simulink model "mc_sevcong4s10"  (R2025a)
settings: Solver=FixedStepAuto  StartTime=0.0  StopTime=10.0  FixedStep=0.05  RelTol=1e-3
settings Model: Creator=adam  LastModifiedBy=adam

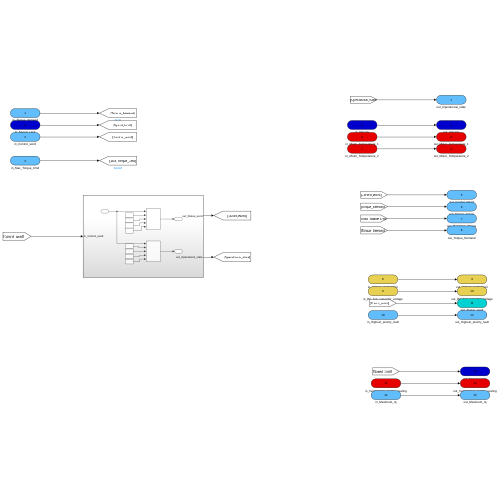
[thumbnail: Simulink's stored preview of the top-level diagram]
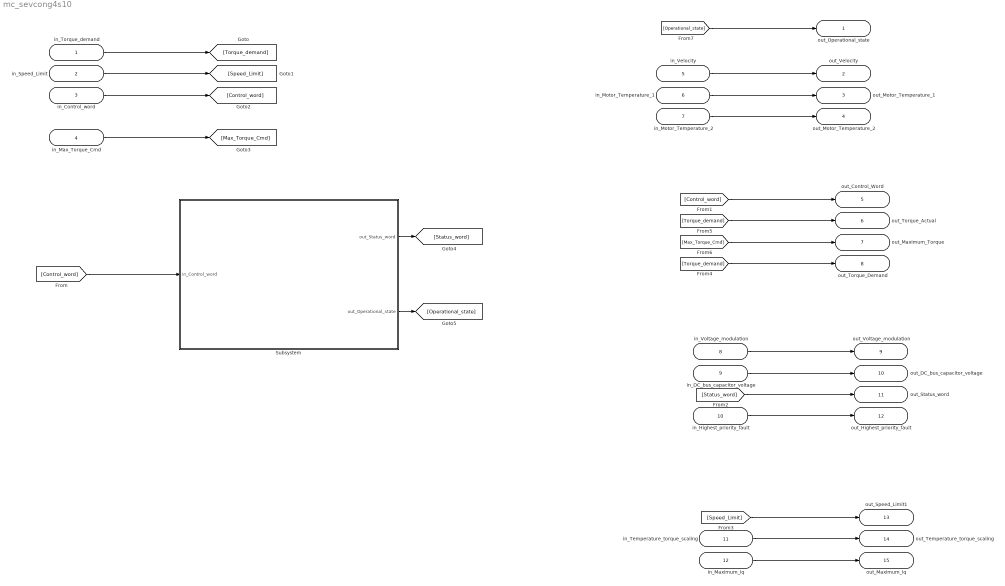
== system mc_sevcong4s10 ==
  in_Torque_demand : Inport
  in_Speed_Limit : Inport  Port=2
  in_Control_word : Inport  Port=3
  in_Max_Torque_Cmd : Inport  Port=4
  in_Velocity : Inport  Port=5
  in_Motor_Temperature_1 : Inport  Port=6
  in_Motor_Temperature_2 : Inport  Port=7
  in_Voltage_modulation : Inport  Port=8
  in_DC_bus_capacitor_voltage : Inport  Port=9
  in_Highest_priority_fault : Inport  Port=10
  in_Temperature_torque_scaling : Inport  Port=11
  in_Maximum_Iq : Inport  Port=12
  Subsystem : Subsystem
  out_Operational_state : Outport
  out_Velocity : Outport  Port=2
  out_Motor_Temperature_1 : Outport  Port=3
  out_Motor_Temperature_2 : Outport  Port=4
  out_Control_Word : Outport  Port=5
  out_Torque_Actual : Outport  Port=6
  out_Maximum_Torque : Outport  Port=7
  out_Torque_Demand : Outport  Port=8
  out_Voltage_modulation : Outport  Port=9
  out_DC_bus_capacitor_voltage : Outport  Port=10
  out_Status_word : Outport  Port=11
  out_Highest_priority_fault : Outport  Port=12
  out_Speed_Limit1 : Outport  Port=13
  out_Temperature_torque_scaling : Outport  Port=14
  out_Maximum_Iq : Outport  Port=15
  wires:
  in_Torque_demand/1 -> [Torque_demand]
  in_Speed_Limit/1 -> [Speed_Limit]
  in_Control_word/1 -> [Control_word]
  in_Max_Torque_Cmd/1 -> [Max_Torque_Cmd]
  [Operational_state] -> out_Operational_state/1
  in_Motor_Temperature_2/1 -> out_Motor_Temperature_2/1
  in_Velocity/1 -> out_Velocity/1
  in_Motor_Temperature_1/1 -> out_Motor_Temperature_1/1
  [Max_Torque_Cmd] -> out_Maximum_Torque/1
  [Torque_demand] -> out_Torque_Actual/1
  [Control_word] -> out_Control_Word/1
  [Torque_demand] -> out_Torque_Demand/1
  in_DC_bus_capacitor_voltage/1 -> out_DC_bus_capacitor_voltage/1
  in_Voltage_modulation/1 -> out_Voltage_modulation/1
  [Status_word] -> out_Status_word/1
  in_Highest_priority_fault/1 -> out_Highest_priority_fault/1
  in_Maximum_Iq/1 -> out_Maximum_Iq/1
  in_Temperature_torque_scaling/1 -> out_Temperature_torque_scaling/1
  [Speed_Limit] -> out_Speed_Limit1/1
  [Control_word] -> Subsystem/1(in_Control_word)
  Subsystem/1(out_Status_word) -> [Status_word]
  Subsystem/2(out_Operational_state) -> [Operational_state]

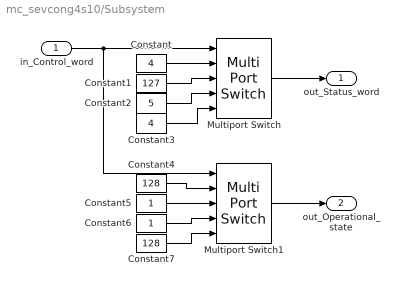
== system mc_sevcong4s10/Subsystem ==
  in_Control_word : Inport
  Constant : Constant  Value=4
  Constant1 : Constant  Value=127
  Constant2 : Constant  Value=5
  Constant3 : Constant  Value=4
  Constant4 : Constant  Value=128
  Constant5 : Constant
  Constant6 : Constant
  Constant7 : Constant  Value=128
  Multiport Switch : MultiPortSwitch  DataPortOrder=Specify indices  DataPortIndices={6,7,15}  DataPortForDefault=Additional data port  DiagnosticForDefault=None  SaturateOnIntegerOverflow=off  InputSameDT=off
  Multiport Switch1 : MultiPortSwitch  DataPortOrder=Specify indices  DataPortIndices={6,7,15}  DataPortForDefault=Additional data port  DiagnosticForDefault=None  SaturateOnIntegerOverflow=off  InputSameDT=off
  out_Status_word : Outport
  out_Operational_state : Outport  Port=2
  wires:
  Multiport Switch/1 -> out_Status_word/1
  Constant/1 -> Multiport Switch/2
  Constant1/1 -> Multiport Switch/3
  Constant2/1 -> Multiport Switch/4
  Constant3/1 -> Multiport Switch/5
  Constant4/1 -> Multiport Switch1/2
  Constant7/1 -> Multiport Switch1/5
  Multiport Switch1/1 -> out_Operational_state/1
  Constant6/1 -> Multiport Switch1/4
  in_Control_word/1 -> Multiport Switch1/1, Multiport Switch/1
  Constant5/1 -> Multiport Switch1/3
